simulink model "main_sim_adapt_Gref_SP"  (Simulink 7.2)
settings: Solver=ode2  SolverMode=SingleTasking  StartTime=0.0  StopTime=tsim_max  FixedStep=dtsim  RelTol=1e-3
StopFcn:
  | %mkplt
values from neighbouring files (symbols this model uses):
  aero_surf_qbar_off = get_value('aero_surf_qbar_off')    [setup_claw.m]
  aero_surf_qbar_on = get_value('aero_surf_qbar_on')    [setup_claw.m]
  assertion_time = get_value('assertion_time')    [setup_sim.m]
  att_cmd_select = get_value('att_cmd_select')    [setup_sim.m]
  att_trim_IC = orientation.att'    [setup_claw.m]
  att_type_numbers = cell2mat(struct2cell(att_type))    [setup_constants.m]
  chi_trim_IC = orientation.Vchigam(2)    [setup_claw.m]
  command_time = engage_time + 2.0    [setup_sim.m]
  compute_all_rate_cols = get_value('compute_all_rate_cols')    [setup_claw.m]
  compute_all_vel_cols = get_value('compute_all_vel_cols')    [setup_claw.m]
  da_trim_IC = tmp(1)    [setup_claw.m]
  dc_L2W_IC = orientation.dc_L2W    [setup_claw.m]
  de_trim_IC = tmp(2)    [setup_claw.m]
  dr_trim_IC = tmp(3)    [setup_claw.m]
  dtsim = get_value('dtsim')    [setup_sim.m]
  E_trim_IC = MACH_pos_IC(2)    [setup_claw.m]
  Ed_trim_IC = MACH_vel_IC(2)    [setup_claw.m]
  gain_set = gain_set_next    (= 1)    [setup_claw.m]
  gain_var_struct = rmfield(gain_var_struct,setdiff(fieldnames(gain_var_struct),{'name','size'}))    [setup_claw.m]
  gamma_trim_IC = orientation.Vchigam(3)    [setup_claw.m]
  h_trim_IC = MACH_pos_IC(3)    [setup_claw.m]
  hd_trim_IC = MACH_vel_IC(3)    [setup_claw.m]
  ideal_vel_Kb = MACH_vel_Kb(1)    [setup_sim.m]
  MACH = rmfield(MACH,'vel_throt_lrlim')    [setup_claw.m]
  MACH_att_fb = get_value('MACH_att_fb','onerror',0)    [setup_claw.m]
  MACH_att_int_IC = (1-MACH_att_Kc).*MACH_quat_IC'    [setup_ideal.m]
  MACH_att_Kb = repval(att_kbnom,MACH.att_num_cv)    [setup_claw.m]
  MACH_att_Kc = Ki2Kc(MACH_att_Ki)    [setup_ideal.m]
  MACH_att_Ki = repval(att_fi,MACH.att_num_cv)    [setup_claw.m]
  MACH_gain_mat = vertcat(MACH_gain_mat, this_gain_mat)    [setup_claw.m]
  MACH_mass_IC = obac_params.mass_IC    [setup_claw.m]
  MACH_pos_IC = x_obac_IC(MACH.NEh_idx)    [setup_claw.m]
  MACH_pos_int_IC = (1-MACH_pos_Kc).*MACH_pos_IC' + MACH_vel_IC'./MACH_pos_Kb    [setup_ideal.m]
  MACH_pos_Kb = repval(pos_kbnom,MACH.pos_num_cv)    [setup_claw.m]
  MACH_pos_Kc = Ki2Kc(MACH_pos_Ki)    [setup_ideal.m]
  MACH_pos_Ki = repval(pos_fi,MACH.pos_num_cv)    [setup_claw.m]
  MACH_pqr_Bmat_IC = Bo(MACH.pqr_idx,MACH.pqr_u_idx)    [setup_claw.m]
  MACH_pqr_IC = pqr_trim_IC    [setup_claw.m]
  MACH_pqr_int_IC = (1-MACH_pqr_Kc).*MACH_pqr_IC'    [setup_ideal.m]
  MACH_pqr_Kb = repval(pqr_kbnom,MACH.pqr_num_cv)    [setup_claw.m]
  MACH_pqr_Kc = Ki2Kc(MACH_pqr_Ki)    [setup_ideal.m]
  MACH_pqr_Ki = repval(pqr_fi,MACH.pqr_num_cv)    [setup_claw.m]
  MACH_pqr_u_IC = [ vanes_trim_IC; tvc_trim_IC; rcs_trim_IC ]    [setup_claw.m]
  MACH_quat_IC = quat_trim_IC    [setup_claw.m]
  MACH_throttle_IC = throttle_trim_IC    [setup_claw.m]
  MACH_U_nom_IC = zeros(MACH.num_u,1)    [setup_claw.m]
  MACH_vel_Bmat_IC = MACH_vel_Bmat_IC*inv(vel_perts)    [setup_claw.m]
  MACH_vel_cvdnom_IC = repval(get_value('vel_cvdnom_IC','onerror',MACH_vel_cvdnom_IC),length(MACH_vel_cvdnom_IC))'    [setup_claw.m]
  MACH_vel_IC = orientation.NdEdhd'    [setup_claw.m]
  MACH_vel_int_IC = (1-MACH_vel_Kc).*MACH_vel_IC'    [setup_ideal.m]
  MACH_vel_Kb = repval(vel_kbnom,MACH.vel_num_cv)    [setup_claw.m]
  MACH_vel_Kc = Ki2Kc(MACH_vel_Ki)    [setup_ideal.m]
  MACH_vel_Ki = repval(vel_fi,MACH.vel_num_cv)    [setup_claw.m]
  MACH_vel_uold_IC = [ MACH_quat_IC; MACH_throttle_IC ]    [setup_claw.m]
  N_trim_IC = MACH_pos_IC(1)    [setup_claw.m]
  Nd_trim_IC = MACH_vel_IC(1)    [setup_claw.m]
  obac_params = define_model('obac', get_value('obac_model_type'))    [setup_claw.m]
  pos_cmd_select = get_value('pos_cmd_select')    [setup_sim.m]
  pqr_trim_IC = [ 0 0 0 ]'    [setup_claw.m]
  rate_cmd_select = get_value('rate_cmd_select')    [setup_sim.m]
  rcs_cvddes_thresh = get_value('rcs_cvddes_thresh')    [setup_claw.m]
  reset_camcmd_on_entry = get_value('reset_camcmd_on_entry')    [setup_claw.m]
  throttle_trim_IC = u_obac_IC(MACH.throttle_idx)    [setup_claw.m]
  trac_params = define_model('trac', get_value('trac_model_type','onerror',obac_params.model_type))    [setup_sim.m]
  use_auto_att_type = get_value('use_auto_att_type','onerror',0)    [setup_claw.m]
  use_eow_as_iv = get_value('use_eow_as_iv')    [setup_claw.m]
  use_full_surf_cmd = get_value('use_full_surf_cmd')    [setup_sim.m]
  use_nav = get_value('use_nav')    [setup_claw.m]
  use_NdEdh_pos = get_value('use_NdEdh_pos')    [setup_claw.m]
  use_pos_fltpath_lim = get_value('use_pos_fltpath_lim')    [setup_claw.m]
  use_throt_estimate = get_value('use_throt_estimate')    [setup_claw.m]
  use_variable_mass = get_value('use_variable_mass')    [setup_claw.m]
  use_wind_est = get_value('use_wind_est')    [setup_claw.m]
  V_trim_IC = orientation.Vchigam(1)    [setup_claw.m]
  vel_cmd_ramp_time = get_value('vel_cmd_ramp_time')    [setup_claw.m]
  vel_cmd_select = get_value('vel_cmd_select')    [setup_sim.m]
  x_trac_IC = x_obac_IC    [setup_sim.m]
undefined symbols (not defined in the file or in its folder): accel_cmd, alpha_trim, Am, att_type, B1, bb_ellipsoid, bb_params, Bm, C, constants, cosA, DiscIntNeverNeededParam, DZkx, DZtheta, E_rwy, Ed_cmd, eow_boundary, flag_autoadapt, flag_exsig, flag_uad, full_surf_llim, full_surf_ulim, gam_cmd_descent, gam_cmd_preflare, gamdot_cmd_descent, gamdot_cmd_flare, gamdot_cmd_preflare, Gamtheta, Gamx, hd_cmd, in_error_thresh, in_exsig_vecin, in_exsig_vecout, in_reset_stoptime, in_t_exsig, in_t_timer, in_tadaptoff_forced, in_tadapton_forced, Kb, Kxhat0, Kxnom, Kxstar, max_chi_cmd, max_LOS_rate, max_vel_cmd, min_chi_cmd, min_vel_cmd, modes, N_rwy, Nd_cmd, Nrbf, P, pos, Sig, sinA, target_pos_IC, target_range_blind, target_range_detect, target_range_homing, target_vel_IC ... (+11)
libraries: simulink x44, utility_lib x36, mach_lib x24, model_lib x13, simulink_need_slupdate x8, models x8
(part 7 of 8)

== system main_sim_adapt_Gref_SP/control input (modified)/ideal responses/ideal pos vel response/get posvel cmd ==
  control_input : Inport  OutDataType=sfix(16)  OutScaling=2^0
  Bus Selector : BusSelector  OutputSignals=mode_sw.CLAW_mode,command
  Constant1 : Constant  Value=MACH_vel_IC  OutDataType=sfix(16)  OutScaling=2^0
  Constant2 : Constant  Value=[4 5 6]  OutDataType=sfix(16)  OutScaling=2^0
  Constant3 : Constant  Value=[4 5 3]  OutDataType=sfix(16)  OutScaling=2^0
  Constant4 : Constant  Value=[1 2 3]  OutDataType=sfix(16)  OutScaling=2^0
  Constant5 : Constant  Value=[1 2 3]  OutDataType=sfix(16)  OutScaling=2^0
  Constant6 : Constant  Value=[4 5 6]  OutDataType=sfix(16)  OutScaling=2^0
  Constant7 : Constant  Value=[1 2 6]  OutDataType=sfix(16)  OutScaling=2^0
  Multiport Switch : MultiPortSwitch  Inputs=6  zeroidx=on
  Multiport Switch1 : MultiPortSwitch  Inputs=6  zeroidx=on
  Multiport Switch2 : MultiPortSwitch  Inputs=6  zeroidx=on
  Selector : Selector  InputPortWidth=4  IndexOptions=Index vector (dialog)  Indices=[1 2 4]  OutputSizes=1
  Switch : Switch  Threshold=0.5
  Switch1 : Switch  Threshold=0.5
  use_full_surf_cmd_sw : Constant  Value=use_NdEdh_pos  OutDataType=sfix(16)  OutScaling=2^0
  use_full_surf_cmd_sw1 : Constant  Value=use_NdEdh_pos  OutDataType=sfix(16)  OutScaling=2^0
  posvel_cmd : Outport  OutDataType=sfix(16)  OutScaling=2^0
  pos_select : Outport  Port=2  OutDataType=sfix(16)  OutScaling=2^0
  vel_select : Outport  Port=3  OutDataType=sfix(16)  OutScaling=2^0
  wires:
  Multiport Switch/1 -> posvel_cmd/1
  Bus Selector/1 -> Multiport Switch/1, Multiport Switch1/1, Multiport Switch2/1  "<CLAW_mode>"
  control_input/1 -> Bus Selector/1
  Constant1/1 -> Multiport Switch/2, Multiport Switch/3, Multiport Switch/4
  Selector/1 -> Multiport Switch/5, Multiport Switch/6, Multiport Switch/7
  Multiport Switch1/1 -> pos_select/1
  Multiport Switch2/1 -> vel_select/1
  Constant2/1 -> Multiport Switch1/2, Multiport Switch1/3, Multiport Switch1/4, Multiport Switch1/5
  Switch/1 -> Multiport Switch1/6
  Constant4/1 -> Multiport Switch2/2, Multiport Switch2/3, Multiport Switch2/4, Multiport Switch2/5
  Constant5/1 -> Multiport Switch1/7, Switch/3
  Constant6/1 -> Multiport Switch2/7, Switch1/3
  Switch1/1 -> Multiport Switch2/6
  Bus Selector/2 -> Selector/1  "<command>"
  use_full_surf_cmd_sw/1 -> Switch/2
  Constant3/1 -> Switch/1
  Constant7/1 -> Switch1/1
  use_full_surf_cmd_sw1/1 -> Switch1/2

== system main_sim_adapt_Gref_SP/control input (modified)/ideal responses/ideal pos vel response/pos loop ==
  NEh_cmd : Inport  OutDataType=sfix(16)  OutScaling=2^0
  NEh : Inport  Port=2  OutDataType=sfix(16)  OutScaling=2^0
  Discrete-Time Integrator : DiscreteIntegrator  IntegratorMethod=Integration: Backward Euler  InitialCondition=MACH_pos_int_IC  SampleTime=-1  OutDataType=sfix(16)  OutScaling=2^0  ICPrevOutput=DiscIntNeverNeededParam  ICPrevScaledInput=DiscIntNeverNeededParam
  Gain1 : Gain  Gain=MACH_pos_Kb  ParameterDataType=sfix(16)  ParameterScaling=2^0  OutDataType=sfix(16)  OutScaling=2^0  SaturateOnIntegerOverflow=on  OutDataTypeStr=Inherit: Same as input  ParamDataTypeStr=Inherit: Same as input
  Gain4 : Gain  Gain=MACH_pos_Kc  ParameterDataType=sfix(16)  ParameterScaling=2^0  OutDataType=sfix(16)  OutScaling=2^0  SaturateOnIntegerOverflow=on  OutDataTypeStr=Inherit: Same as input  ParamDataTypeStr=Inherit: Same as input
  Gain5 : Gain  Gain=MACH_pos_Ki.*MACH_pos_Kb  ParameterDataType=sfix(16)  ParameterScaling=2^0  OutDataType=sfix(16)  OutScaling=2^0  SaturateOnIntegerOverflow=on  OutDataTypeStr=Inherit: Same as input  ParamDataTypeStr=Inherit: Same as input
  Sum2 : Sum  Inputs=|+-  OutDataType=sfix(16)  OutScaling=2^0  SaturateOnIntegerOverflow=on  InputSameDT=on  OutDataTypeStr=Inherit: Same as first input
  Sum3 : Sum  Inputs=++-  OutDataType=sfix(16)  OutScaling=2^0  SaturateOnIntegerOverflow=on  InputSameDT=on  OutDataTypeStr=Inherit: Same as first input
  NEhdot_cmd : Outport  OutDataType=sfix(16)  OutScaling=2^0
  wires:
  Sum2/1 -> Gain5/1
  Sum3/1 -> Gain1/1
  Gain4/1 -> Sum3/1
  Discrete-Time Integrator/1 -> Sum3/2
  Gain5/1 -> Discrete-Time Integrator/1
  Gain1/1 -> NEhdot_cmd/1
  NEh_cmd/1 -> Sum2/1, Gain4/1
  NEh/1 -> Sum2/2, Sum3/3

== system main_sim_adapt_Gref_SP/control input (modified)/ideal responses/ideal pos vel response/vel loop ==
  NEhdot_cmd : Inport  OutDataType=sfix(16)  OutScaling=2^0
  NEhdot : Inport  Port=2  OutDataType=sfix(16)  OutScaling=2^0
  Discrete-Time Integrator1 : DiscreteIntegrator  IntegratorMethod=Integration: Backward Euler  InitialCondition=MACH_vel_int_IC  SampleTime=-1  OutDataType=sfix(16)  OutScaling=2^0  ICPrevOutput=DiscIntNeverNeededParam  ICPrevScaledInput=DiscIntNeverNeededParam
  Gain : Gain  Gain=MACH_vel_Kb  ParameterDataType=sfix(16)  ParameterScaling=2^0  OutDataType=sfix(16)  OutScaling=2^0  SaturateOnIntegerOverflow=on  OutDataTypeStr=Inherit: Same as input  ParamDataTypeStr=Inherit: Same as input
  Gain2 : Gain  Gain=MACH_vel_Kc  ParameterDataType=sfix(16)  ParameterScaling=2^0  OutDataType=sfix(16)  OutScaling=2^0  SaturateOnIntegerOverflow=on  OutDataTypeStr=Inherit: Same as input  ParamDataTypeStr=Inherit: Same as input
  Gain3 : Gain  Gain=MACH_vel_Ki.*MACH_vel_Kb  ParameterDataType=sfix(16)  ParameterScaling=2^0  OutDataType=sfix(16)  OutScaling=2^0  SaturateOnIntegerOverflow=on  OutDataTypeStr=Inherit: Same as input  ParamDataTypeStr=Inherit: Same as input
  Sum : Sum  Inputs=|+-  OutDataType=sfix(16)  OutScaling=2^0  SaturateOnIntegerOverflow=on  InputSameDT=on  OutDataTypeStr=Inherit: Same as first input
  Sum1 : Sum  Inputs=++-  OutDataType=sfix(16)  OutScaling=2^0  SaturateOnIntegerOverflow=on  InputSameDT=on  OutDataTypeStr=Inherit: Same as first input
  NEhdotdot : Outport  OutDataType=sfix(16)  OutScaling=2^0
  wires:
  Sum/1 -> Gain3/1
  NEhdot_cmd/1 -> Gain2/1, Sum/1
  Gain/1 -> NEhdotdot/1
  Sum1/1 -> Gain/1
  Gain2/1 -> Sum1/1
  Discrete-Time Integrator1/1 -> Sum1/2
  Gain3/1 -> Discrete-Time Integrator1/1
  NEhdot/1 -> Sum/2, Sum1/3

== system main_sim_adapt_Gref_SP/vehicle_model/target/seeker model/seeker model/cart to polar ==
  note: Avoid division by zero when
      | all errors are exactly zero
  scaling info : Inport  OutDataType=sfix(16)  OutScaling=2^0
  cross_d;vert_d : Inport  Port=2  OutDataType=sfix(16)  OutScaling=2^0
  Abs : Abs
  Bus Selector : BusSelector  OutputSignals=Rground,Rslant
  Constant : Constant  Value=0.0001  OutDataType=sfix(16)  OutScaling=2^0
  Gain1 : Gain  Gain=1./max_LOS_rate  ParameterDataType=sfix(16)  ParameterScaling=2^0  OutDataType=sfix(16)  OutScaling=2^0
  Gain2 : Gain  Gain=[1 -1]  ParameterDataType=sfix(16)  ParameterScaling=2^0  OutDataType=sfix(16)  OutScaling=2^0
  MinMax : MinMax  Function=max  Inputs=3  OutDataType=sfix(16)  OutScaling=2^0
  Mux : Mux  Inputs=2
  Product : Product  Inputs=*/  OutDataType=sfix(16)  OutScaling=2^0  RndMeth=Zero
  LOS_rate : Outport  OutDataType=sfix(16)  OutScaling=2^0
  wires:
  Mux/1 -> MinMax/2
  Gain1/1 -> MinMax/1
  Gain2/1 -> Product/2
  MinMax/1 -> Gain2/1
  Abs/1 -> Gain1/1
  Product/1 -> LOS_rate/1
  cross_d;vert_d/1 -> Product/1, Abs/1
  scaling info/1 -> Bus Selector/1
  Bus Selector/1 -> Mux/1  "<Rground>"
  Bus Selector/2 -> Mux/2  "<Rslant>"
  Constant/1 -> MinMax/3

== system main_sim_adapt_Gref_SP/claw_main/input processing/mode dependent stick processing/att rate cmd/also reset att on att_type change ==
  reset_in : Inport  OutDataType=sfix(16)  OutScaling=2^0
  Detect Change : simulink/Logic and Bit Operations/Detect Change  SystemSampleTime=-1  vinit=0
  Detect Increase : simulink/Logic and Bit Operations/Detect Increase  SystemSampleTime=-1  vinit=0.0
  Logical Operator2 : Logic  Operator=OR  AllPortsSameDT=off
  Logical Operator3 : Logic  Operator=XOR  AllPortsSameDT=off
  Unit Delay : UnitDelay  Orientation=left  SampleTime=MACH.dt
  reset_out : Outport  OutDataType=sfix(16)  OutScaling=2^0
  wires:
  [att_type] -> Detect Change/1
  Detect Change/1 -> Logical Operator2/2
  Detect Increase/1 -> Logical Operator2/1
  Logical Operator2/1 -> Logical Operator3/1
  Logical Operator3/1 -> Unit Delay/1, reset_out/1
  Unit Delay/1 -> Logical Operator3/2
  reset_in/1 -> Detect Increase/1

== system main_sim_adapt_Gref_SP/claw_main/input processing/mode dependent stick processing/feed forward/get att_ff ==
  signal_bus : Inport  OutDataType=sfix(16)  OutScaling=2^0
  Bus Selector : BusSelector  OutputSignals=x_est.uvw,y_meas.accels_cg,y_meas.dircos,x_est.e
  Dot Product : simulink/Math Operations/Dot Product  InputSameDT=on  OutDataType=sfix(16)  OutScaling=2^-10  DoSatur=off
  Gain : Gain  Gain=constants.g  ParameterDataType=sfix(16)  ParameterScaling=2^0  OutDataType=sfix(16)  OutScaling=2^0
  MinMax1 : MinMax  Function=max  Inputs=2  OutDataType=sfix(16)  OutScaling=2^0
  Product1 : Product  Inputs=/*  OutDataType=sfix(16)  OutScaling=2^0  RndMeth=Zero
  Sum2 : Sum  Inputs=|++  OutDataType=sfix(16)  OutScaling=2^0
  V x a : utility_lib/cross product  SystemSampleTime=-1
  down vector : Selector  InputPortWidth=9  IndexOptions=Index vector (dialog)  Indices=7:9  OutputSizes=1
  geted : utility_lib/geted  SystemSampleTime=-1
  protect for   divide by zero : Constant  Value=0.001^2  OutDataType=sfix(16)  OutScaling=2^0
  att_ff : Outport  OutDataType=sfix(16)  OutScaling=2^0
  wires:
  Product1/1 -> geted/1
  V x a/1 -> Product1/2
  signal_bus/1 -> Bus Selector/1
  Bus Selector/1 -> V x a/1, Dot Product/1, Dot Product/2  "<uvw>"
  Bus Selector/4 -> geted/2  "<e>"
  protect for   divide by zero/1 -> MinMax1/2
  MinMax1/1 -> Product1/1
  Sum2/1 -> V x a/2
  geted/1 -> att_ff/1
  Bus Selector/3 -> down vector/1  "<dircos>"
  down vector/1 -> Gain/1
  Gain/1 -> Sum2/2
  Bus Selector/2 -> Sum2/1  "<accels_cg>"
  Dot Product/1 -> MinMax1/1

== system main_sim_adapt_Gref_SP/claw_main/input processing/mode dependent stick processing/feed forward/lookup using  energy over weight ==
  eow_idx : Inport  OutDataType=sfix(16)  OutScaling=2^0
  Constant1 : Constant  Value=int32(0:2)  OutDataType=sfix(16)  OutScaling=2^0
  Constant2 : Constant  Value=int32(0:2)  OutDataType=sfix(16)  OutScaling=2^0
  Interpolation (n-D) using PreLookup for acc : simulink_need_slupdate/Interpolation (n-D) using PreLookup  numDimsPopupSelect=2  explicitNumDims=2  table=tbl_acc_eow  interpMethod=Linear  extrapMethod=Linear  rangeErrorMode=None  NumSelectionDims=1
  Interpolation (n-D) using PreLookup for vel : simulink_need_slupdate/Interpolation (n-D) using PreLookup  numDimsPopupSelect=2  explicitNumDims=2  table=tbl_vel_eow  interpMethod=Linear  extrapMethod=Linear  rangeErrorMode=None  NumSelectionDims=1
  pos_ff : Outport  OutDataType=sfix(16)  OutScaling=2^0
  vel_ff : Outport  Port=2  OutDataType=sfix(16)  OutScaling=2^0
  wires:
  Interpolation (n-D) using PreLookup for vel/1 -> pos_ff/1
  Interpolation (n-D) using PreLookup for acc/1 -> vel_ff/1
  eow_idx/1 -> Interpolation (n-D) using PreLookup for vel/1, Interpolation (n-D) using PreLookup for acc/1
  Constant1/1 -> Interpolation (n-D) using PreLookup for vel/2
  Constant2/1 -> Interpolation (n-D) using PreLookup for acc/2

== system main_sim_adapt_Gref_SP/claw_main/input processing/mode dependent stick processing/feed forward/lookup using X   ==
  X_idx : Inport  OutDataType=sfix(16)  OutScaling=2^0
  Constant1 : Constant  Value=int32(0:2)  OutDataType=sfix(16)  OutScaling=2^0
  Constant2 : Constant  Value=int32(0:2)  OutDataType=sfix(16)  OutScaling=2^0
  Interpolation (n-D) using PreLookup for acc : simulink_need_slupdate/Interpolation (n-D) using PreLookup  numDimsPopupSelect=2  explicitNumDims=2  table=tbl_acc_X  interpMethod=Linear  extrapMethod=Linear  rangeErrorMode=None  NumSelectionDims=1
  Interpolation (n-D) using PreLookup for vel : simulink_need_slupdate/Interpolation (n-D) using PreLookup  numDimsPopupSelect=2  explicitNumDims=2  table=tbl_vel_X  interpMethod=Linear  extrapMethod=Linear  rangeErrorMode=None  NumSelectionDims=1
  pos_ff : Outport  OutDataType=sfix(16)  OutScaling=2^0
  vel_ff : Outport  Port=2  OutDataType=sfix(16)  OutScaling=2^0
  wires:
  X_idx/1 -> Interpolation (n-D) using PreLookup for vel/1, Interpolation (n-D) using PreLookup for acc/1
  Interpolation (n-D) using PreLookup for vel/1 -> pos_ff/1
  Interpolation (n-D) using PreLookup for acc/1 -> vel_ff/1
  Constant1/1 -> Interpolation (n-D) using PreLookup for vel/2
  Constant2/1 -> Interpolation (n-D) using PreLookup for acc/2

== system main_sim_adapt_Gref_SP/claw_main/input processing/mode dependent stick processing/set command selection switches/modify for accel cmd submode ==
  select_cmd_in : Inport  OutDataType=sfix(16)  OutScaling=2^0
  accel_cmd_sw : Inport  Port=2  OutDataType=sfix(16)  OutScaling=2^0
  Assignment : Assignment  IndexOptions=Index vector (dialog)  Indices=[1 2 4]  OutputSizes=[1 1]
  Assignment1 : Assignment  IndexOptions=Index vector (dialog)  Indices=[1 2 4]  OutputSizes=[1 1]
  Bus Assignment : BusAssignment  AssignedSignals=vel,pos
  Bus Selector : BusSelector  OutputSignals=vel
  Bus Selector1 : BusSelector  OutputSignals=pos
  Selector1 : Selector  InputPortWidth=4  IndexOptions=Index vector (dialog)  Indices=[1 2 4]  OutputSizes=1
  Selector2 : Selector  InputPortWidth=4  IndexOptions=Index vector (dialog)  Indices=[1 2 4]  OutputSizes=1
  Switch : Switch  Threshold=0.5
  Switch1 : Switch  Threshold=0.5
  command current pos : Constant  Value=0  OutDataType=sfix(16)  OutScaling=2^0
  command current vel : Constant  Value=0  OutDataType=sfix(16)  OutScaling=2^0
  select_cmd : Outport  OutDataType=sfix(16)  OutScaling=2^0
  wires:
  select_cmd_in/1 -> Bus Assignment/1, Bus Selector/1, Bus Selector1/1
  accel_cmd_sw/1 -> Switch/2, Switch1/2
  Bus Selector/1 -> Selector1/1, Assignment/1  "<vel>"
  command current vel/1 -> Switch/1
  Selector1/1 -> Switch/3
  Switch/1 -> Assignment/2
  Assignment/1 -> Bus Assignment/2
  Bus Assignment/1 -> select_cmd/1
  Bus Selector1/1 -> Selector2/1, Assignment1/1  "<pos>"
  command current pos/1 -> Switch1/1
  Selector2/1 -> Switch1/3
  Switch1/1 -> Assignment1/2
  Assignment1/1 -> Bus Assignment/3

== system main_sim_adapt_Gref_SP/claw_main/input processing/mode dependent stick processing/use table lookup pos cmds/use E/W to get pos cmds ==
  eow_idx : Inport  OutDataType=sfix(16)  OutScaling=2^0
  Constant1 : Constant  Value=int32(0:2)  OutDataType=sfix(16)  OutScaling=2^0
  Interpolation (n-D) using PreLookup : simulink_need_slupdate/Interpolation (n-D) using PreLookup  numDimsPopupSelect=2  explicitNumDims=2  table=tbl_pos_eow  interpMethod=Linear  extrapMethod=Linear  rangeErrorMode=None  NumSelectionDims=1
  pos_cmd_eow : Outport  OutDataType=sfix(16)  OutScaling=2^0
  wires:
  Interpolation (n-D) using PreLookup/1 -> pos_cmd_eow/1
  eow_idx/1 -> Interpolation (n-D) using PreLookup/1
  Constant1/1 -> Interpolation (n-D) using PreLookup/2

== system main_sim_adapt_Gref_SP/claw_main/input processing/mode dependent stick processing/use table lookup pos cmds/use X to get pos cmds ==
  note: Note: When X is used as the independent variable
      | the trajectory is in a vertical plane and Y=0
  X_idx : Inport  OutDataType=sfix(16)  OutScaling=2^0
  X : Inport  Port=2  OutDataType=sfix(16)  OutScaling=2^0
  Constant1 : Constant  Value=E_rwy  OutDataType=sfix(16)  OutScaling=2^0
  Constant3 : Constant  Value=N_rwy  OutDataType=sfix(16)  OutScaling=2^0
  Constant4 : Constant  Value=cosA  OutDataType=sfix(16)  OutScaling=2^0
  Constant5 : Constant  Value=sinA  OutDataType=sfix(16)  OutScaling=2^0
  Interpolation (n-D) using PreLookup for h : simulink_need_slupdate/Interpolation (n-D) using PreLookup  numDimsPopupSelect=1  explicitNumDims=2  table=tbl_hofX  interpMethod=Linear  extrapMethod=Linear  rangeErrorMode=None  NumSelectionDims=0
  Mux : Mux  Inputs=3
  Product3 : Product  OutDataType=sfix(16)  OutScaling=2^0  RndMeth=Zero
  Product4 : Product  OutDataType=sfix(16)  OutScaling=2^0  RndMeth=Zero
  Sum4 : Sum  Inputs=++|  OutDataType=sfix(16)  OutScaling=2^0
  Sum5 : Sum  Inputs=|++  OutDataType=sfix(16)  OutScaling=2^0
  pos_cmd_X : Outport  OutDataType=sfix(16)  OutScaling=2^0
  wires:
  X_idx/1 -> Interpolation (n-D) using PreLookup for h/1
  Interpolation (n-D) using PreLookup for h/1 -> Mux/3
  Mux/1 -> pos_cmd_X/1
  Constant4/1 -> Product4/1
  Constant5/1 -> Product3/1
  Sum4/1 -> Mux/1
  Product4/1 -> Sum4/2
  Constant3/1 -> Sum4/1
  Sum5/1 -> Mux/2
  Product3/1 -> Sum5/1
  Constant1/1 -> Sum5/2
  X/1 -> Product4/2, Product3/2

== system main_sim_adapt_Gref_SP/claw_main/input processing/set control parameters/accel submode setup/NED_dd/vchigam_dot ==
  case : Inport  OutDataType=sfix(16)  OutScaling=2^0
  signal_bus : Inport  Port=2  OutDataType=sfix(16)  OutScaling=2^0
  Action Port : ActionPort  ActionType=case
  Bus Selector3 : BusSelector  OutputSignals=cmd_bus.autopilot_cmd
  Gain : Gain  Gain=[1 1 1]  ParameterDataType=sfix(16)  ParameterScaling=2^0  OutDataType=sfix(16)  OutScaling=2^0
  Selector : Selector  InputPortWidth=4  IndexOptions=Index vector (dialog)  Indices=[1 2 4]  OutputSizes=1
  Signal Conversion : SignalConversion  ConversionOutput=Contiguous copy
  accel_cmd_sw : Outport  OutDataType=sfix(16)  OutScaling=2^0  InitialOutput=zeros(3,1)
  accel_cmd : Outport  Port=2  OutDataType=sfix(16)  OutScaling=2^0  InitialOutput=zeros(3,1)
  wires:
  signal_bus/1 -> Bus Selector3/1
  Bus Selector3/1 -> Selector/1  "<autopilot_cmd>"
  Selector/1 -> Signal Conversion/1
  case/1 -> Gain/1
  Gain/1 -> accel_cmd_sw/1
  Signal Conversion/1 -> accel_cmd/1

== system main_sim_adapt_Gref_SP/claw_main/input processing/set control parameters/accel submode setup/homing ==
  signal_bus : Inport  OutDataType=sfix(16)  OutScaling=2^0
  Action Port : ActionPort  ActionType=case
  Bus Selector3 : BusSelector  OutputSignals=y_meas.seeker.aux_info.Rslant,y_meas.seeker.LOS_rate
  Compare To Constant : simulink/Logic and Bit Operations/Compare To Constant  SystemSampleTime=-1  relop=<=  const=target_range_homing  LogicOutDataTypeMode=boolean  ZeroCross=off
  Compare To Constant1 : simulink/Logic and Bit Operations/Compare To Constant  SystemSampleTime=-1  relop=<=  const=target_range_detect  LogicOutDataTypeMode=boolean  ZeroCross=off
  Compare To Constant2 : simulink/Logic and Bit Operations/Compare To Constant  SystemSampleTime=-1  relop=>=  const=target_range_blind  LogicOutDataTypeMode=boolean  ZeroCross=off
  Constant2 : Constant  Value=0  OutDataType=sfix(16)  OutScaling=2^0
  Data Type Conversion : DataTypeConversion  OutDataTypeMode=double  OutDataType=sfix(16)  OutScaling=2^0  OutDataTypeStr=double
  Gain : Gain  Gain=2  ParameterDataType=sfix(16)  ParameterScaling=2^0  OutDataType=sfix(16)  OutScaling=2^0  OutDataTypeStr=Inherit: Inherit via back propagation
  Logical Operator2 : Logic  AllPortsSameDT=off
  Mux : Mux  Inputs=2
  Mux1 : Mux  Inputs=2
  Product3 : Product  OutDataType=sfix(16)  OutScaling=2^0  RndMeth=Zero
  Selector3 : Selector  InputPortWidth=2  IndexOptions=Index vector (dialog)  Indices=[1 1 2]  OutputSizes=1
  azimuth_d/elevation_d gain : Gain  Gain=MACH.K_pn  ParameterDataType=sfix(16)  ParameterScaling=2^0  OutDataType=sfix(16)  OutScaling=2^0
  accel_cmd_sw : Outport  OutDataType=sfix(16)  OutScaling=2^0  InitialOutput=zeros(3,1)
  accel_cmd : Outport  Port=2  OutDataType=sfix(16)  OutScaling=2^0  InitialOutput=zeros(3,1)
  wires:
  Bus Selector3/1 -> Compare To Constant/1, Compare To Constant1/1, Compare To Constant2/1  "<Rslant>"
  Compare To Constant1/1 -> Mux/1
  Compare To Constant/1 -> Mux/2
  Mux/1 -> Logical Operator2/1, Selector3/1
  Compare To Constant2/1 -> Logical Operator2/2
  Selector3/1 -> Data Type Conversion/1
  signal_bus/1 -> Bus Selector3/1
  Bus Selector3/2 -> Product3/2  "<LOS_rate>"
  Product3/1 -> azimuth_d/elevation_d gain/1
  Logical Operator2/1 -> Product3/1  "PN_active"
  Constant2/1 -> Mux1/1
  azimuth_d/elevation_d gain/1 -> Mux1/2
  Gain/1 -> accel_cmd_sw/1
  Mux1/1 -> accel_cmd/1
  Data Type Conversion/1 -> Gain/1

== system main_sim_adapt_Gref_SP/claw_main/input processing/set control parameters/accel submode setup/normal vel desdyn ==
  Action Port : ActionPort  ActionType=default
  Constant1 : Constant  Value=zeros(3,1)  OutDataType=sfix(16)  OutScaling=2^0
  Constant2 : Constant  Value=zeros(3,1)  OutDataType=sfix(16)  OutScaling=2^0
  accel_cmd_sw : Outport  OutDataType=sfix(16)  OutScaling=2^0  InitialOutput=zeros(3,1)
  accel_cmd : Outport  Port=2  OutDataType=sfix(16)  OutScaling=2^0  InitialOutput=zeros(3,1)
  wires:
  Constant1/1 -> accel_cmd/1
  Constant2/1 -> accel_cmd_sw/1

== system main_sim_adapt_Gref_SP/claw_main/input processing/set control parameters/select gains/mux to bus ==
  mux_in : Inport  OutDataType=sfix(16)  OutScaling=2^0
  Bus Creator : BusCreator  Inputs=16
  Demux : Demux  Outputs=[4;4;4;4;3;3;3;3;3;3;3;3;3;3;3;3]
  bus_out : Outport  OutDataType=sfix(16)  OutScaling=2^0
  wires:
  mux_in/1 -> Demux/1
  Bus Creator/1 -> bus_out/1
  Demux/1 -> Bus Creator/1  "MACH_att_Kaw"
  Demux/2 -> Bus Creator/2  "MACH_att_Kb"
  Demux/3 -> Bus Creator/3  "MACH_att_Kf"
  Demux/4 -> Bus Creator/4  "MACH_att_Ki"
  Demux/5 -> Bus Creator/5  "MACH_pos_Kaw"
  Demux/6 -> Bus Creator/6  "MACH_pos_Kb"
  Demux/7 -> Bus Creator/7  "MACH_pos_Kf"
  Demux/8 -> Bus Creator/8  "MACH_pos_Ki"
  Demux/9 -> Bus Creator/9  "MACH_pqr_Kaw"
  Demux/10 -> Bus Creator/10  "MACH_pqr_Kb"
  Demux/11 -> Bus Creator/11  "MACH_pqr_Kf"
  Demux/12 -> Bus Creator/12  "MACH_pqr_Ki"
  Demux/13 -> Bus Creator/13  "MACH_vel_Kaw"
  Demux/14 -> Bus Creator/14  "MACH_vel_Kb"
  Demux/15 -> Bus Creator/15  "MACH_vel_Kf"
  Demux/16 -> Bus Creator/16  "MACH_vel_Ki"

== system main_sim_adapt_Gref_SP/claw_main/input processing/set control parameters/set rate di params/fix aero surfs when low qbar ==
  pqr_u_ulim_in : Inport  OutDataType=sfix(16)  OutScaling=2^0
  pqr_u_llim_in : Inport  Port=2  OutDataType=sfix(16)  OutScaling=2^0
  low_qbar : Inport  Port=3  OutDataType=sfix(16)  OutScaling=2^0
  pqr_u_pref : Inport  Port=4  OutDataType=sfix(16)  OutScaling=2^0
  Assignment : Assignment  IndexOptions=Index vector (dialog)  Indices=MACH.vane_idx  OutputSizes=[1 1]
  Assignment1 : Assignment  IndexOptions=Index vector (dialog)  Indices=MACH.vane_idx  OutputSizes=[1 1]
  MinMax : MinMax  Inputs=2  OutDataType=sfix(16)  OutScaling=2^0
  MinMax1 : MinMax  Function=max  Inputs=2  OutDataType=sfix(16)  OutScaling=2^0
  Multiport Switch1 : MultiPortSwitch  Inputs=2  zeroidx=on  SaturateOnIntegerOverflow=on
  Multiport Switch2 : MultiPortSwitch  Inputs=2  zeroidx=on  SaturateOnIntegerOverflow=on
  Selector1 : Selector  InputPortWidth=MACH.pqr_num_u  IndexOptions=Index vector (dialog)  Indices=MACH.vane_idx  OutputSizes=1
  Selector2 : Selector  InputPortWidth=MACH.pqr_num_u  IndexOptions=Index vector (dialog)  Indices=MACH.vane_idx  OutputSizes=1
  Selector6 : Selector  InputPortWidth=MACH.pqr_num_u  IndexOptions=Index vector (dialog)  Indices=MACH.vane_idx  OutputSizes=1
  pqr_u_ulim : Outport  OutDataType=sfix(16)  OutScaling=2^0
  pqr_u_llim : Outport  Port=2  OutDataType=sfix(16)  OutScaling=2^0
  wires:
  low_qbar/1 -> Multiport Switch1/1, Multiport Switch2/1
  pqr_u_pref/1 -> Selector6/1
  pqr_u_ulim_in/1 -> Assignment/1, Multiport Switch1/2, Selector1/1
  pqr_u_llim_in/1 -> Assignment1/1, Multiport Switch2/2, Selector2/1
  Multiport Switch1/1 -> pqr_u_ulim/1
  Assignment/1 -> Multiport Switch1/3
  Multiport Switch2/1 -> pqr_u_llim/1
  Assignment1/1 -> Multiport Switch2/3
  Selector1/1 -> MinMax/1
  Selector6/1 -> MinMax/2
  MinMax/1 -> MinMax1/1
  Selector2/1 -> MinMax1/2
  MinMax1/1 -> Assignment/2, Assignment1/2

== system main_sim_adapt_Gref_SP/claw_main/input processing/set control parameters/set rate di params/select u_pref ==
  note: "from outer" not yet implemented
  note: "test" not yet implemented
  note: Use schedule if configured and qbar is low
  low_qbar : Inport  OutDataType=sfix(16)  OutScaling=2^0
  aero_env_est : Inport  Port=2  OutDataType=sfix(16)  OutScaling=2^0
  full_surf : Inport  Port=3  OutDataType=sfix(16)  OutScaling=2^0
  Bus Selector4 : BusSelector  OutputSignals=full_surf_pref_select,full_surf_pref,full_surf_pref_wght,full_surf_cmd
  Constant2 : Constant  Value=MACH.pqr_wght_u_pref_high  OutDataType=sfix(16)  OutScaling=2^0
  Demux : Demux  Outputs=2
  From Workspace : FromWorkspace  VariableName=use_preference_schedule_fw  SampleTime=MACH.dt  Interpolate=off  OutputAfterFinalValue=Holding final value
  Logical Operator : Logic  AllPortsSameDT=off
  Logical Operator1 : Logic  Operator=NOT  AllPortsSameDT=off
  MinMax : MinMax  Function=max  Inputs=2  OutDataType=sfix(16)  OutScaling=2^0
  Multiport Switch : MultiPortSwitch  Inputs=5  zeroidx=on
  Mux{,1..3} (4 alike) : Mux  Inputs=2
  Selector{1..3,5} (4 alike) : Selector  InputPortWidth=MACH.num_u  IndexOptions=Index vector (dialog)  Indices=MACH.pqr_u_idx  OutputSizes=1
  preference schedule : model_lib/no preference schedule  SystemSampleTime=-1
  u_pref : Outport  OutDataType=sfix(16)  OutScaling=2^0
  wght_u_pref : Outport  Port=2  OutDataType=sfix(16)  OutScaling=2^0
  wires:
  Selector1/1 -> preference schedule/1, Mux/1
  Selector2/1 -> preference schedule/2, Mux/2
  Mux/1 -> Multiport Switch/2, Multiport Switch/5, Multiport Switch/6
  Multiport Switch/1 -> Demux/1
  Demux/1 -> u_pref/1
  Demux/2 -> wght_u_pref/1
  aero_env_est/1 -> preference schedule/3
  preference schedule/1 -> Mux1/1
  preference schedule/2 -> Mux1/2
  Mux1/1 -> Multiport Switch/3
  low_qbar/1 -> Logical Operator1/1
  full_surf/1 -> Bus Selector4/1
  Mux2/1 -> Multiport Switch/4
  Constant2/1 -> Mux2/2
  Selector5/1 -> Mux2/1
  Bus Selector4/1 -> Selector3/1  "<full_surf_pref_select>"
  Bus Selector4/2 -> Selector1/1  "<full_surf_pref>"
  Bus Selector4/3 -> Selector2/1  "<full_surf_pref_wght>"
  Bus Selector4/4 -> Selector5/1  "<full_surf_cmd>"
  Selector3/1 -> MinMax/2
  Mux3/1 -> Multiport Switch/1
  MinMax/1 -> Mux3/1, Mux3/2
  Logical Operator1/1 -> Logical Operator/2
  From Workspace/1 -> Logical Operator/1
  Logical Operator/1 -> MinMax/1

== system main_sim_adapt_Gref_SP/claw_main/state est/wind estimator/wind estimate/rate and  position limits ==
  w_est : Inport  OutDataType=sfix(16)  OutScaling=2^0
  Constant : Constant  Value=MACH.est_w_ulim  OutDataType=sfix(16)  OutScaling=2^0
  Constant1 : Constant  Value=MACH.est_w_llim  OutDataType=sfix(16)  OutScaling=2^0
  Constant2 : Constant  Value=MACH.est_w_urlim  OutDataType=sfix(16)  OutScaling=2^0
  Constant3 : Constant  Value=MACH.est_w_lrlim  OutDataType=sfix(16)  OutScaling=2^0
  MinMax : MinMax  Function=max  Inputs=2  OutDataType=sfix(16)  OutScaling=2^0  SaturateOnIntegerOverflow=on  InputSameDT=on
  MinMax1 : MinMax  Inputs=2  OutDataType=sfix(16)  OutScaling=2^0  SaturateOnIntegerOverflow=on  InputSameDT=on
  Unit Delay : UnitDelay  SampleTime=-1
  limit computation : mach_lib/limit computation  SystemSampleTime=-1
  w_est_lim : Outport  OutDataType=sfix(16)  OutScaling=2^0
  wires:
  w_est/1 -> MinMax1/1
  Unit Delay/1 -> limit computation/1
  MinMax1/1 -> MinMax/1
  limit computation/1 -> MinMax1/2
  Constant/1 -> limit computation/3
  Constant1/1 -> limit computation/2
  Constant2/1 -> limit computation/4
  MinMax/1 -> w_est_lim/1, Unit Delay/1
  limit computation/2 -> MinMax/2
  Constant3/1 -> limit computation/5

== system main_sim_adapt_Gref_SP/claw_main/vel_loops/B matrix comp/B matrix comp/compute cvd_pert ==
  note: Note: this computation of NEh accelerations
      | assumes that pqr = 0
  x : Inport  OutDataType=sfix(16)  OutScaling=2^0
  u : Inport  Port=2  OutDataType=sfix(16)  OutScaling=2^0
  w_est : Inport  Port=3  OutDataType=sfix(16)  OutScaling=2^0
  Bus Selector : BusSelector  OutputSignals=dircos
  Gain : Gain  Gain=[1 1 -1]  ParameterDataType=sfix(16)  ParameterScaling=2^0  OutDataType=sfix(16)  OutScaling=2^0  SaturateOnIntegerOverflow=on  OutDataTypeStr=Inherit: Same as input  ParamDataTypeStr=Inherit: Same as input
  Math Function : Math  Operator=transpose  OutDataType=sfix(16)  OutScaling=2^0  SaturateOnIntegerOverflow=on
  Product : Product  Multiplication=Matrix(*)  OutDataType=sfix(16)  OutScaling=2^0  SaturateOnIntegerOverflow=on  InputSameDT=on  OutDataTypeStr=Inherit: Same as first input
  Reshape : Reshape  OutputDimensionality=Customize  OutputDimensions=[3,3]
  cl model : models/gtm-obac  SystemSampleTime=-1
  uvw_dot : Selector  InputPortWidth=MACH.num_x  IndexOptions=Index vector (dialog)  Indices=MACH.uvw_idx  OutputSizes=1
  cvd : Outport  OutDataType=sfix(16)  OutScaling=2^0
  wires:
  uvw_dot/1 -> Product/2
  x/1 -> cl model/1
  Reshape/1 -> Math Function/1
  Math Function/1 -> Product/1
  Product/1 -> Gain/1
  Gain/1 -> cvd/1
  Bus Selector/1 -> Reshape/1  "<dircos>"
  u/1 -> cl model/2
  w_est/1 -> cl model/3
  cl model/1 -> uvw_dot/1
  cl model/2 -> Bus Selector/1

== system main_sim_adapt_Gref_SP/claw_main/vel_loops/B matrix comp/B matrix comp/compute perturbed XU ==
  X_in : Inport  OutDataType=sfix(16)  OutScaling=2^0
  U_in : Inport  Port=2  OutDataType=sfix(16)  OutScaling=2^0
  D_in : Inport  Port=3  OutDataType=sfix(16)  OutScaling=2^0
  camcmd : Inport  Port=4  OutDataType=sfix(16)  OutScaling=2^0
  NEh_dot : Inport  Port=5  OutDataType=sfix(16)  OutScaling=2^0
  Assignment1 : Assignment  IndexOptions=Index vector (dialog)  Indices=MACH.throttle_idx  OutputSizes=[1 1]
  Assignment2 : Assignment  IndexOptions=Index vector (dialog)  Indices=[ MACH.quat_idx MACH.uvw_idx]  OutputSizes=[1 1]
  Demux1 : Demux  Outputs=[ 2 MACH.num_u_throt ]
  Gain : Gain  Gain=[1 1 -1]  ParameterDataType=sfix(16)  ParameterScaling=2^0  OutDataType=sfix(16)  OutScaling=2^0  SaturateOnIntegerOverflow=on  OutDataTypeStr=Inherit: Same as input  ParamDataTypeStr=Inherit: Same as input
  Mux : Mux  Inputs=[ 2 1 ]
  Mux1 : Mux  Inputs=2
  Product1 : Product  Multiplication=Matrix(*)  OutDataType=sfix(16)  OutScaling=2^0  SaturateOnIntegerOverflow=on  OutDataTypeStr=Inherit: Same as first input
  Reshape1 : Reshape  OutputDimensionality=Customize  OutputDimensions=[3,3]
  Selector1 : Selector  InputPortWidth=MACH.num_x  IndexOptions=Index vector (dialog)  Indices=MACH.quat_idx  OutputSizes=1
  att2dc : utility_lib/att2dc  SystemSampleTime=-1
  dc2e_ref : utility_lib/dc2e_ref  SystemSampleTime=-1
  X_out : Outport  OutDataType=sfix(16)  OutScaling=2^0
  U_out : Outport  Port=2  OutDataType=sfix(16)  OutScaling=2^0
  wires:
  Mux/1 -> att2dc/1
  Demux1/2 -> Assignment1/2  "throttle"
  D_in/1 -> Demux1/1
  U_in/1 -> Assignment1/1
  X_in/1 -> Assignment2/1, Selector1/1
  Assignment1/1 -> U_out/1
  camcmd/1 -> Mux/2
  Demux1/1 -> Mux/1
  NEh_dot/1 -> Gain/1
  Reshape1/1 -> Product1/1
  Assignment2/1 -> X_out/1
  att2dc/1 -> Reshape1/1, dc2e_ref/1
  dc2e_ref/1 -> Mux1/1  "e"
  Gain/1 -> Product1/2  "NED_dot"
  Selector1/1 -> dc2e_ref/2
  Product1/1 -> Mux1/2  "uvw"
  Mux1/1 -> Assignment2/2

== system main_sim_adapt_Gref_SP/claw_main/vel_loops/B matrix comp/B matrix comp/pert_comp ==
  col : Inport  OutDataType=sfix(16)  OutScaling=2^0
  d_nom : Inport  Port=2  OutDataType=sfix(16)  OutScaling=2^0
  params : Inport  Port=3  OutDataType=sfix(16)  OutScaling=2^0
  Bus Selector : BusSelector  OutputSignals=u_ulim,u_llim
  Constant2 : Constant  Value=diag(MACH.vel_u_pert)  OutDataType=sfix(16)  OutScaling=2^0
  pick +/- pert : mach_lib/pick +//- pert  SystemSampleTime=-1  num_u=MACH.vel_num_u
  d_pert : Outport  OutDataType=sfix(16)  OutScaling=2^0
  d_div : Outport  Port=2  OutDataType=sfix(16)  OutScaling=2^0
  wires:
  pick +/- pert/2 -> d_div/1  "scalar pert value"
  d_nom/1 -> pick +/- pert/2
  pick +/- pert/1 -> d_pert/1
  col/1 -> pick +/- pert/1
  Constant2/1 -> pick +/- pert/5
  params/1 -> Bus Selector/1
  Bus Selector/1 -> pick +/- pert/3  "<u_ulim>"
  Bus Selector/2 -> pick +/- pert/4  "<u_llim>"

== system main_sim_adapt_Gref_SP/claw_main/vel_loops/convert accel_cmd to NED_dd_cmd/vchigam_dot cmd/polar to cart ==
  note: Note: these are actually Vground and Vslant
  scaling_info : Inport  OutDataType=sfix(16)  OutScaling=2^0
  vchigam_dot_cmd : Inport  Port=2  OutDataType=sfix(16)  OutScaling=2^0
  Bus Selector : BusSelector  OutputSignals=Rground,Rslant
  Demux : Demux  Outputs=[1 2]
  Gain1 : Gain  Gain=[1 -1]  ParameterDataType=sfix(16)  ParameterScaling=2^0  OutDataType=sfix(16)  OutScaling=2^0
  Mux : Mux  Inputs=2
  Mux1 : Mux  Inputs=2
  Product3 : Product  OutDataType=sfix(16)  OutScaling=2^0  RndMeth=Zero
  along_dd;cross_dd;vert_dd : Outport  OutDataType=sfix(16)  OutScaling=2^0
  wires:
  scaling_info/1 -> Bus Selector/1
  Mux/1 -> Gain1/1
  vchigam_dot_cmd/1 -> Demux/1
  Bus Selector/1 -> Mux/1  "<Rground>"
  Bus Selector/2 -> Mux/2  "<Rslant>"
  Gain1/1 -> Product3/2
  Demux/2 -> Product3/1
  Demux/1 -> Mux1/1
  Product3/1 -> Mux1/2
  Mux1/1 -> along_dd;cross_dd;vert_dd/1

== system main_sim_adapt_Gref_SP/control input (modified)/control input/form control input/select command/att cmd select ==
  cmd_bus : Inport  OutDataType=sfix(16)  OutScaling=2^0
  Bus Selector1 : BusSelector  OutputSignals=att1_cmd,att2_cmd,att3_cmd,throttle_cmd  OutputAsBus=on
  Bus Selector2 : BusSelector  OutputSignals=att_cmd
  Switch : Switch  Threshold=0.5
  use_cam_rate_cmd1 : Constant  Value=att_cmd_select  OutDataType=sfix(16)  OutScaling=2^0
  att_cmd : Outport  OutDataType=sfix(16)  OutScaling=2^0
  wires:
  Bus Selector1/1 -> Switch/3
  Bus Selector2/1 -> Switch/1  "<att_cmd>"
  cmd_bus/1 -> Bus Selector1/1, Bus Selector2/1
  use_cam_rate_cmd1/1 -> Switch/2
  Switch/1 -> att_cmd/1

== system main_sim_adapt_Gref_SP/control input (modified)/control input/form control input/select command/pos cmd select ==
  cmd_bus : Inport  OutDataType=sfix(16)  OutScaling=2^0
  Bus Selector1 : BusSelector  OutputSignals=N_cmd,E_cmd,att3_cmd,h_cmd  OutputAsBus=on
  Bus Selector3 : BusSelector  OutputSignals=pos_cmd,accel_submode
  Bus Selector5 : BusSelector  OutputSignals=Vd_cmd,chid_cmd,att3_cmd,gammad_cmd  OutputAsBus=on
  Bus Selector6 : BusSelector  OutputSignals=Ndd_cmd,Edd_cmd,att3_cmd,hdd_cmd  OutputAsBus=on
  Constant : Constant  Value=use_NdEdh_pos  OutDataType=sfix(16)  OutScaling=2^0
  Ground : Ground
  Multiport Switch : MultiPortSwitch  Inputs=2  zeroidx=on
  Multiport Switch1 : MultiPortSwitch  Inputs=4  zeroidx=on
  Switch : Switch  Threshold=0.5
  convert if use_Vchigam : Subsystem
  use_cam_rate_cmd1 : Constant  Value=pos_cmd_select  OutDataType=sfix(16)  OutScaling=2^0
  pos_cmd : Outport  OutDataType=sfix(16)  OutScaling=2^0
  wires:
  Constant/1 -> Multiport Switch/1
  convert if use_Vchigam/1(pos_cmd) -> Multiport Switch/3
  Bus Selector1/1 -> Multiport Switch/2
  cmd_bus/1 -> Bus Selector1/1, Bus Selector6/1, Bus Selector5/1, convert if use_Vchigam/1(cmd_bus), Bus Selector3/1
  use_cam_rate_cmd1/1 -> Switch/2
  Switch/1 -> pos_cmd/1
  Bus Selector3/1 -> Switch/1  "<pos_cmd>"
  Bus Selector3/2 -> Multiport Switch1/1  "<accel_submode>"
  Multiport Switch/1 -> Multiport Switch1/2
  Ground/1 -> Multiport Switch1/5
  Bus Selector6/1 -> Multiport Switch1/3
  Bus Selector5/1 -> Multiport Switch1/4
  Multiport Switch1/1 -> Switch/3

== system main_sim_adapt_Gref_SP/control input (modified)/control input/form control input/select command/rate cmd select ==
  cmd_bus : Inport  OutDataType=sfix(16)  OutScaling=2^0
  Bus Selector1 : BusSelector  OutputSignals=p_cmd,q_cmd,r_cmd,throttle_cmd  OutputAsBus=on
  Bus Selector3 : BusSelector  OutputSignals=rate_cmd  OutputAsBus=on
  Switch : Switch  Threshold=0.5
  use_cam_rate_cmd1 : Constant  Value=rate_cmd_select  OutDataType=sfix(16)  OutScaling=2^0
  rate_cmd : Outport  OutDataType=sfix(16)  OutScaling=2^0
  wires:
  Switch/1 -> rate_cmd/1
  use_cam_rate_cmd1/1 -> Switch/2
  cmd_bus/1 -> Bus Selector3/1, Bus Selector1/1
  Bus Selector3/1 -> Switch/1
  Bus Selector1/1 -> Switch/3

== system main_sim_adapt_Gref_SP/control input (modified)/control input/form control input/select command/vel cmd select ==
  cmd_bus : Inport  OutDataType=sfix(16)  OutScaling=2^0
  Bus Selector1 : BusSelector  OutputSignals=Vd_cmd,chid_cmd,att3_cmd,gammad_cmd  OutputAsBus=on
  Bus Selector2 : BusSelector  OutputSignals=vel_cmd,accel_submode
  Bus Selector4 : BusSelector  OutputSignals=Ndd_cmd,Edd_cmd,att3_cmd,hdd_cmd  OutputAsBus=on
  Ground : Ground
  Multiport Switch : MultiPortSwitch  Inputs=4  zeroidx=on
  Switch : Switch  Threshold=0.5
  convert if use_Vchigam : Subsystem
  use_cam_rate_cmd1 : Constant  Value=vel_cmd_select  OutDataType=sfix(16)  OutScaling=2^0
  vel_cmd : Outport  OutDataType=sfix(16)  OutScaling=2^0
  wires:
  Switch/1 -> vel_cmd/1
  use_cam_rate_cmd1/1 -> Switch/2
  cmd_bus/1 -> Bus Selector2/1, Bus Selector4/1, Bus Selector1/1, convert if use_Vchigam/1(cmd_bus)
  Bus Selector2/1 -> Switch/1  "<vel_cmd>"
  Bus Selector2/2 -> Multiport Switch/1  "<accel_submode>"
  Bus Selector4/1 -> Multiport Switch/3
  Ground/1 -> Multiport Switch/5
  Bus Selector1/1 -> Multiport Switch/4
  Multiport Switch/1 -> Switch/3
  convert if use_Vchigam/1(vel_cmd) -> Multiport Switch/2

== system main_sim_adapt_Gref_SP/control input (modified)/control input/generate commands/pos cmd generator/circle pos cmd ==
  cmd_bus : Inport  OutDataType=sfix(16)  OutScaling=2^0
  Bus Selector1 : BusSelector  OutputSignals=att3_cmd,h_cmd  OutputAsBus=on
  Constant : Constant  OutDataType=sfix(16)  OutScaling=2^0
  Gain : Gain  Gain=50  ParameterDataType=sfix(16)  ParameterScaling=2^0  OutDataType=sfix(16)  OutScaling=2^0
  Gain1 : Gain  Gain=50  ParameterDataType=sfix(16)  ParameterScaling=2^0  OutDataType=sfix(16)  OutScaling=2^0
  Gain2 : Gain  Gain=0.1  ParameterDataType=sfix(16)  ParameterScaling=2^0  OutDataType=sfix(16)  OutScaling=2^0
  Gain3 : Gain  ParameterDataType=sfix(16)  ParameterScaling=2^0  OutDataType=sfix(16)  OutScaling=2^0
  Mux1 : Mux  Inputs=3
  Ramp : Subsystem  mask{slope=1, start_time=command_time, initial_output=0, sample_time=MACH.dt}
      mask prompts: start_time "Start time:"; initial_output "Initial output:"; sample_time "Sample time (-1 for inherited):"
  Saturation1 : Saturate  UpperLimit=10  LowerLimit=0
  Sum : Sum  Inputs=|-+  OutDataType=sfix(16)  OutScaling=2^0
  Sum1 : Sum  Inputs=++|  OutDataType=sfix(16)  OutScaling=2^0
  Sum2 : Sum  Inputs=-+|  OutDataType=sfix(16)  OutScaling=2^0
  Trigonometric Function : Trigonometry
  Trigonometric Function1 : Trigonometry  Operator=cos
  pos_cmd : Outport  OutDataType=sfix(16)  OutScaling=2^0
  wires:
  Sum/1 -> Gain1/1
  Trigonometric Function/1 -> Gain/1
  Sum2/1 -> Gain2/1
  Trigonometric Function1/1 -> Sum/1
  Constant/1 -> Sum/2
  Gain1/1 -> Mux1/2
  Sum1/1 -> Mux1/1
  Gain/1 -> Sum1/2
  Ramp/1(ramp) -> Saturation1/1, Sum2/2
  Saturation1/1 -> Sum2/1, Gain3/1
  Gain2/1 -> Trigonometric Function/1, Trigonometric Function1/1
  Gain3/1 -> Sum1/1
  cmd_bus/1 -> Bus Selector1/1
  Bus Selector1/1 -> Mux1/3
  Mux1/1 -> pos_cmd/1

== system main_sim_adapt_Gref_SP/control input (modified)/control input/generate commands/pos cmd generator/ramp pos cmd ==
  cmd_bus : Inport  OutDataType=sfix(16)  OutScaling=2^0
  Bus Selector1 : BusSelector  OutputSignals=E_cmd,att3_cmd,h_cmd  OutputAsBus=on
  Discrete-Time Integrator1 : DiscreteIntegrator  SampleTime=-1  OutDataType=sfix(16)  OutScaling=2^0  ICPrevOutput=DiscIntNeverNeededParam  ICPrevScaledInput=DiscIntNeverNeededParam
  Discrete-Time Integrator3 : DiscreteIntegrator  SampleTime=-1  OutDataType=sfix(16)  OutScaling=2^0  ICPrevOutput=DiscIntNeverNeededParam  ICPrevScaledInput=DiscIntNeverNeededParam
  Gain : Gain  Gain=ideal_vel_Kb  ParameterDataType=sfix(16)  ParameterScaling=2^0  OutDataType=sfix(16)  OutScaling=2^0
  Mux : Mux  Inputs=2
  Sum6 : Sum  Inputs=|+-  OutDataType=sfix(16)  OutScaling=2^0  SaturateOnIntegerOverflow=on
  limit acceleration to g/3 : Saturate  UpperLimit=constants.g/3  LowerLimit=-constants.g/3
  velocity command : Step  Time=command_time  After=1.69*15  SampleTime=MACH.dt
  pos_cmd : Outport  OutDataType=sfix(16)  OutScaling=2^0
  wires:
  limit acceleration to g/3/1 -> Discrete-Time Integrator3/1
  Gain/1 -> limit acceleration to g/3/1
  Sum6/1 -> Gain/1
  velocity command/1 -> Sum6/1
  Discrete-Time Integrator3/1 -> Discrete-Time Integrator1/1, Sum6/2
  Discrete-Time Integrator1/1 -> Mux/1
  Mux/1 -> pos_cmd/1
  cmd_bus/1 -> Bus Selector1/1
  Bus Selector1/1 -> Mux/2

== system main_sim_adapt_Gref_SP/control input (modified)/control input/generate commands/vel cmd generator/Ramp ==
  From Workspace1 : FromWorkspace  VariableName=[ 0 initial_output ; start_time initial_output ; start_time+1 initial_output+slope ]  SampleTime=MACH.dt
  ramp : Outport  OutDataType=sfix(16)  OutScaling=2^0
  wires:
  From Workspace1/1 -> ramp/1

== system main_sim_adapt_Gref_SP/control input (modified)/control input/generate commands/vel cmd generator/descent ==
  From Workspace1 : FromWorkspace  VariableName=[ 0 initial_output ; start_time initial_output ; start_time+1 initial_output+slope ]  SampleTime=MACH.dt
  ramp : Outport  OutDataType=sfix(16)  OutScaling=2^0
  wires:
  From Workspace1/1 -> ramp/1

== system main_sim_adapt_Gref_SP/control input (modified)/control input/generate commands/vel cmd generator/flare ==
  From Workspace1 : FromWorkspace  VariableName=[ 0 initial_output ; start_time initial_output ; start_time+1 initial_output+slope ]  SampleTime=MACH.dt
  ramp : Outport  OutDataType=sfix(16)  OutScaling=2^0
  wires:
  From Workspace1/1 -> ramp/1

== system main_sim_adapt_Gref_SP/control input (modified)/control input/generate commands/vel cmd generator/pre-flare ==
  From Workspace1 : FromWorkspace  VariableName=[ 0 initial_output ; start_time initial_output ; start_time+1 initial_output+slope ]  SampleTime=MACH.dt
  ramp : Outport  OutDataType=sfix(16)  OutScaling=2^0
  wires:
  From Workspace1/1 -> ramp/1

== system main_sim_adapt_Gref_SP/control input (modified)/control input/generate commands/vel cmd generator/turn rate ==
  From Workspace1 : FromWorkspace  VariableName=[ 0 initial_output ; start_time initial_output ; start_time+1 initial_output+slope ]  SampleTime=MACH.dt
  ramp : Outport  OutDataType=sfix(16)  OutScaling=2^0
  wires:
  From Workspace1/1 -> ramp/1

== system main_sim_adapt_Gref_SP/control input (modified)/ideal responses/ideal att rate response/get att cmd/convert to quat ==
  att_cmd : Inport  OutDataType=sfix(16)  OutScaling=2^0
  e : Inport  Port=2  OutDataType=sfix(16)  OutScaling=2^0
  Demux : Demux  Outputs=[2 1]
  Discrete-Time Integrator4 : DiscreteIntegrator  IntegratorMethod=Integration: Backward Euler  InitialCondition=att_trim_IC(3)  SampleTime=-1  OutDataType=sfix(16)  OutScaling=2^0  ICPrevOutput=DiscIntNeverNeededParam  ICPrevScaledInput=DiscIntNeverNeededParam
  From Workspace2 : FromWorkspace  VariableName=use_cam_rate_cmd_fw  SampleTime=MACH.dt  Interpolate=off  OutputAfterFinalValue=Holding final value
  Multiport Switch1 : MultiPortSwitch  Inputs=2  zeroidx=on
  Mux2 : Mux  Inputs=2
  Selector : Selector  InputPortWidth=4  IndexOptions=Index vector (dialog)  Indices=[1 2 3]  OutputSizes=1
  att2dc : utility_lib/att2dc  SystemSampleTime=-1
  dc2e_ref : utility_lib/dc2e_ref  SystemSampleTime=-1
  e_cmd : Outport  OutDataType=sfix(16)  OutScaling=2^0
  wires:
  From Workspace2/1 -> Multiport Switch1/1
  Discrete-Time Integrator4/1 -> Multiport Switch1/3
  Demux/2 -> Multiport Switch1/2, Discrete-Time Integrator4/1
  Multiport Switch1/1 -> Mux2/2
  Demux/1 -> Mux2/1
  att_cmd/1 -> Selector/1
  Selector/1 -> Demux/1
  att2dc/1 -> dc2e_ref/1
  e/1 -> dc2e_ref/2
  Mux2/1 -> att2dc/1
  dc2e_ref/1 -> e_cmd/1
